simulink model "modeloparaIdentificationToolbox"  (R2021a)
settings: Solver=FixedStepAuto  StartTime=0.0  StopTime=200  FixedStep=1e-4  RelTol=1e-3
settings Model: Creator=Royer  LastModifiedBy=Royer

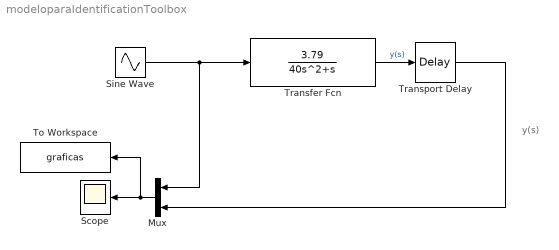
== system modeloparaIdentificationToolbox ==
  note: y(s)
  Mux : Mux  Inputs=2
  Scope : Scope
  Sine Wave : Sin  SampleTime=0
  To Workspace : ToWorkspace  VariableName=graficas  SaveFormat=Timeseries  SampleTime=-1
  Transfer Fcn : TransferFcn  Numerator=[3.79]  Denominator=[40 1 0]  ParameterTunability=Optimized
  Transport Delay : TransportDelay  DelayTime=2
  wires:
  Transfer Fcn/1 -> Transport Delay/1  "y(s)"
  Sine Wave/1 -> Mux/1, Transfer Fcn/1
  Mux/1 -> To Workspace/1, Scope/1
  Transport Delay/1 -> Mux/2
